simulink subsystem "CtrlEnv_Vehicle_refsub"  (R2023a)
settings: Solver=VariableStepAuto  StartTime=0.0  StopTime=10.0  RelTol=1e-3
undefined symbols (not defined in the file): bevPlant, initial
libraries: fl_lib x28, nesl_utility x11, sdl_lib x1
settings Model: Creator=isaacito  LastModifiedBy=antaeug
settings OptimizationCC: ReuseModelBlockBuffer=off

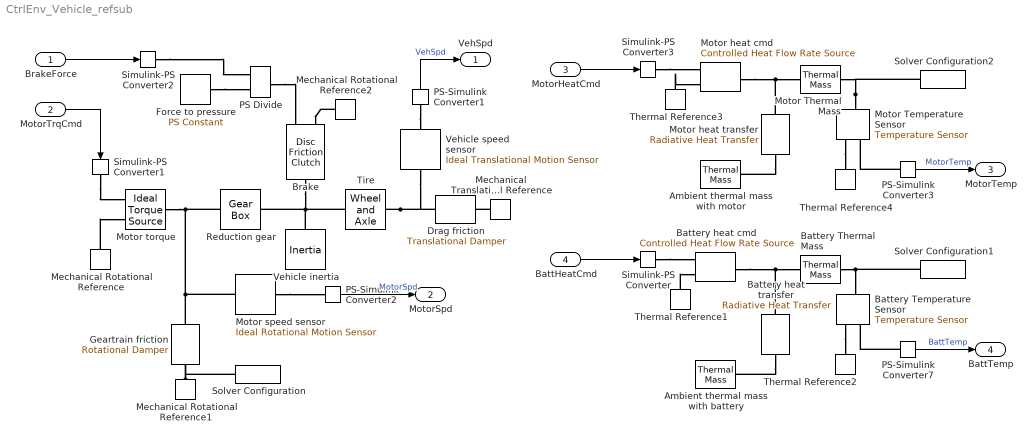
== system CtrlEnv_Vehicle_refsub ==
  BrakeForce : Inport
  MotorTrqCmd : Inport  Port=2
  MotorHeatCmd : Inport  Port=3
  BattHeatCmd : Inport  Port=4
  Ambient thermal mass with battery : fl_lib/Thermal/Thermal Elements/Thermal Mass  mass_type=foundation.enum.constant_variable.constant  mass=1000 t  sp_heat=1000 J/(K*kg)  mass_min=1e-6 kg  num_ports=foundation.enum.numPorts2.one  m_specify=off  m_priority=High  m=1 kg  m_nominal_specify=off  m_nominal_unit=kg  m_nominal_value=1  T_specify=on  T_priority=High  T=initial.BatteryAmbientTemperature_K K  T_nominal_specify=off  T_nominal_unit=K  T_nominal_value=1  Q_specify=off  Q_priority=None  Q=0 W  Q_nominal_specify=off  Q_nominal_unit=W  Q_nominal_value=1
  Ambient thermal mass with motor : fl_lib/Thermal/Thermal Elements/Thermal Mass  mass_type=foundation.enum.constant_variable.constant  mass=1000 t  sp_heat=1000 J/(K*kg)  mass_min=1e-6 kg  num_ports=foundation.enum.numPorts2.one  m_specify=off  m_priority=High  m=1 kg  m_nominal_specify=off  m_nominal_unit=kg  m_nominal_value=1  T_specify=on  T_priority=High  T=initial.MotorAmbientTemperature_K K  T_nominal_specify=off  T_nominal_unit=K  T_nominal_value=1  Q_specify=off  Q_priority=None  Q=0 W  Q_nominal_specify=off  Q_nominal_unit=W  Q_nominal_value=1
  Battery Temperature Sensor : fl_lib/Thermal/Thermal Sensors/Temperature Sensor  temperature_measure=foundation.enum.MeasurementReference.difference
  Battery Thermal Mass : fl_lib/Thermal/Thermal Elements/Thermal Mass  mass_type=foundation.enum.constant_variable.constant  mass=bevPlant.BatteryThermalMass_kg kg  sp_heat=bevPlant.BatterySpecificHeat_J_per_K_per_kg J/(K*kg)  mass_min=1e-6 kg  num_ports=foundation.enum.numPorts2.two  m_specify=off  m_priority=High  m=1 kg  m_nominal_specify=off  m_nominal_unit=kg  m_nominal_value=1  T_specify=on  T_priority=High  T=initial.BatteryTemperature_K K  T_nominal_specify=off  T_nominal_unit=K  T_nominal_value=1  Q_specify=off  Q_priority=None  Q=0 W  Q_nominal_specify=off  Q_nominal_unit=W  Q_nominal_value=1
      settings: InternalSimscapePortConfiguration="{\"Bottom\":[],\"Left\":[{\"id\":\"M\",\"label\":\"\",\"type\":\"foundation.thermal.thermal\"}],\"Right\":[{\"id\":\"N\",\"label\":\"\",\"type\":\"foundation.thermal.thermal\"}],\"Top\":[]}"
  Battery heat cmd : fl_lib/Thermal/Thermal Sources/Controlled Heat Flow Rate Source
  Battery heat transfer : fl_lib/Thermal/Thermal Elements/Radiative Heat Transfer  area=10 m^2  rad_tr_coeff=4e-8 W/(K^4*m^2)  T_specify=off  T_priority=None  T=0 K  T_nominal_specify=off  T_nominal_unit=K  T_nominal_value=1  Q_specify=off  Q_priority=None  Q=0 W  Q_nominal_specify=off  Q_nominal_unit=W  Q_nominal_value=1
      settings: InternalSimscapePortConfiguration="{\"Bottom\":[],\"Left\":[{\"id\":\"A\",\"label\":\"A\",\"type\":\"foundation.thermal.thermal\"}],\"Right\":[{\"id\":\"B\",\"label\":\"B\",\"type\":\"foundation.thermal.thermal\"}],\"Top\":[]}"
  Brake : sdl_lib/Clutches/Disc Friction Clutch  geometry_model=sdl.enum.friction_geometry.radius  r_eff=200 mm  d_o=150 mm  d_i=100 mm  nS=8  piston_area=1 m^2  unidirectional=sdl.enum.directionality.bidirectional  friction_model=sdl.enum.friction_model_TLU_thermal.fixed  mu_w_vector=[0, 100, 1000] rad/s  temperature_TLU=[280, 300, 320] K  mu_static=0.35  mu_static_vector=[.4, .38, .36]  mu_coulomb=0.3  mu_coulomb_vector=[.3, .22, .19]  mu_coulomb_temp_vector=[.3, .28, .25]  mu_coulomb_matrix=[.34, .32, .3; .3, .28, .25; .25, .2, .15]  mu_interp_method=simscape.enum.interpolation.linear  mu_extrap_method=simscape.enum.extrapolation.linear  d_f=1  w_tol=0.001 rad/s  pressure_min=1 Pa  mu_visc=0 N*m*s/rad  initial_state_locked=sdl.enum.initial_lock.unlocked  enable_faults=simscape.enum.onoff.off  fault_type=sdl.enum.clutchFault.lock  external_fault=simscape.enum.onoff.off  temporal_fault=simscape.enum.onoff.off  fault_time=5 s  report_fault=simscape.enum.assert.action.none  thermal_mass=50 kJ/K  T_init=300 K
      settings: InternalSimscapePortConfiguration="{\"Bottom\":[],\"Left\":[{\"id\":\"P\",\"label\":\"P\",\"type\":\"input\"},{\"id\":\"B\",\"label\":\"B\",\"type\":\"foundation.mechanical.rotational.rotational\"}],\"Right\":[{\"id\":\"F\",\"label\":\"F\",\"type\":\"foundation.mechanical.rotational.rotational\"}],\"Top\":[]}"
  Drag friction : fl_lib/Mechanical/Translational Elements/Translational Damper  D=10 N/kph  v_specify=off  v_priority=None  v=0 m/s  v_nominal_specify=off  v_nominal_unit=m/s  v_nominal_value=1  f_specify=off  f_priority=None  f=0 N  f_nominal_specify=off  f_nominal_unit=N  f_nominal_value=1
  Force to pressure : fl_lib/Physical Signals/Sources/PS Constant  constant=1 m^2
  Geartrain friction : fl_lib/Mechanical/Rotational Elements/Rotational Damper  D=0.001 N*m/rpm  w_specify=off  w_priority=None  w=0 rad/s  w_nominal_specify=off  w_nominal_unit=rad/s  w_nominal_value=1  t_specify=off  t_priority=None  t=0 N*m  t_nominal_specify=off  t_nominal_unit=N*m  t_nominal_value=1
  Mechanical Rotational Reference : fl_lib/Mechanical/Rotational Elements/Mechanical Rotational Reference
  Mechanical Rotational Reference1 : fl_lib/Mechanical/Rotational Elements/Mechanical Rotational Reference
  Mechanical Rotational Reference2 : fl_lib/Mechanical/Rotational Elements/Mechanical Rotational Reference
  Mechanical Translational Reference : fl_lib/Mechanical/Translational Elements/Mechanical Translational Reference
  Motor Temperature Sensor : fl_lib/Thermal/Thermal Sensors/Temperature Sensor  temperature_measure=foundation.enum.MeasurementReference.difference
  Motor Thermal Mass : fl_lib/Thermal/Thermal Elements/Thermal Mass  mass_type=foundation.enum.constant_variable.constant  mass=bevPlant.MotorThermalMass_kg kg  sp_heat=bevPlant.MotorSpecificHeat_J_per_K_per_kg J/(K*kg)  mass_min=1e-6 kg  num_ports=foundation.enum.numPorts2.two  m_specify=off  m_priority=High  m=1 kg  m_nominal_specify=off  m_nominal_unit=kg  m_nominal_value=1  T_specify=on  T_priority=High  T=initial.MotorTemperature_K K  T_nominal_specify=off  T_nominal_unit=K  T_nominal_value=1  Q_specify=off  Q_priority=None  Q=0 W  Q_nominal_specify=off  Q_nominal_unit=W  Q_nominal_value=1
      settings: InternalSimscapePortConfiguration="{\"Bottom\":[],\"Left\":[{\"id\":\"M\",\"label\":\"\",\"type\":\"foundation.thermal.thermal\"}],\"Right\":[{\"id\":\"N\",\"label\":\"\",\"type\":\"foundation.thermal.thermal\"}],\"Top\":[]}"
  Motor heat cmd : fl_lib/Thermal/Thermal Sources/Controlled Heat Flow Rate Source
  Motor heat transfer : fl_lib/Thermal/Thermal Elements/Radiative Heat Transfer  area=1 m^2  rad_tr_coeff=4e-8 W/(K^4*m^2)  T_specify=off  T_priority=None  T=0 K  T_nominal_specify=off  T_nominal_unit=K  T_nominal_value=1  Q_specify=off  Q_priority=None  Q=0 W  Q_nominal_specify=off  Q_nominal_unit=W  Q_nominal_value=1
      settings: InternalSimscapePortConfiguration="{\"Bottom\":[],\"Left\":[{\"id\":\"A\",\"label\":\"A\",\"type\":\"foundation.thermal.thermal\"}],\"Right\":[{\"id\":\"B\",\"label\":\"B\",\"type\":\"foundation.thermal.thermal\"}],\"Top\":[]}"
  Motor speed sensor : fl_lib/Mechanical/Mechanical Sensors/Ideal Rotational Motion Sensor  reference=foundation.enum.MeasurementReference.absolute  acceleration_port=false  velocity_port=true  position_port=false  wrap_angle=false  offset=0 rad
      settings: InternalSimscapePortConfiguration="{\"Bottom\":[],\"Left\":[{\"id\":\"R\",\"label\":\"R\",\"type\":\"foundation.mechanical.rotational.rotational\"}],\"Right\":[{\"id\":\"W\",\"label\":\"W\",\"type\":\"output\"}],\"Top\":[]}"
  Motor torque : fl_lib/Mechanical/Mechanical Sources/Ideal Torque Source
  PS Divide : fl_lib/Physical Signals/Functions/PS Divide
  PS-Simulink Converter1 : nesl_utility/PS-Simulink Converter  PhysicalDomain=network_engine_domain  SubClassName=ps_output  LeftPortType=input  RightPortType=output  PseudoPeriodic=off  Frequencies=[]  VectorFormat=inherit  Unit=km/hr  AffineConversion=off
  PS-Simulink Converter2 : nesl_utility/PS-Simulink Converter  PhysicalDomain=network_engine_domain  SubClassName=ps_output  LeftPortType=input  RightPortType=output  PseudoPeriodic=off  Frequencies=[]  VectorFormat=inherit  Unit=rpm  AffineConversion=off
  PS-Simulink Converter3 : nesl_utility/PS-Simulink Converter  PhysicalDomain=network_engine_domain  SubClassName=ps_output  LeftPortType=input  RightPortType=output  PseudoPeriodic=off  Frequencies=[]  VectorFormat=inherit  Unit=degC  AffineConversion=on
  PS-Simulink Converter7 : nesl_utility/PS-Simulink Converter  PhysicalDomain=network_engine_domain  SubClassName=ps_output  LeftPortType=input  RightPortType=output  PseudoPeriodic=off  Frequencies=[]  VectorFormat=inherit  Unit=degC  AffineConversion=on
  Reduction gear : fl_lib/Mechanical/Mechanisms/Gear Box  ratio=bevPlant.ReductionGearRaio  t_in_specify=off  t_in_priority=None  t_in=0 N*m  t_in_nominal_specify=off  t_in_nominal_unit=N*m  t_in_nominal_value=1  t_out_specify=off  t_out_priority=None  t_out=0 N*m  t_out_nominal_specify=off  t_out_nominal_unit=N*m  t_out_nominal_value=1
  Simulink-PS Converter : nesl_utility/Simulink-PS Converter  PhysicalDomain=network_engine_domain  SubClassName=ps_input  LeftPortType=input  RightPortType=output  PseudoPeriodic=off  Frequencies=[]  NoiseDistribution=none  NoiseParameters=[]  Unit=W  AffineConversion=off  FilteringAndDerivatives=provide  SimscapeFilterOrder=1  InputFilterTimeConstant=0.001  UdotUserProvided=0
  Simulink-PS Converter1 : nesl_utility/Simulink-PS Converter  PhysicalDomain=network_engine_domain  SubClassName=ps_input  LeftPortType=input  RightPortType=output  PseudoPeriodic=off  Frequencies=[]  NoiseDistribution=none  NoiseParameters=[]  Unit=N*m  AffineConversion=off  FilteringAndDerivatives=filter  SimscapeFilterOrder=1  InputFilterTimeConstant=0.001  UdotUserProvided=0
  Simulink-PS Converter2 : nesl_utility/Simulink-PS Converter  PhysicalDomain=network_engine_domain  SubClassName=ps_input  LeftPortType=input  RightPortType=output  PseudoPeriodic=off  Frequencies=[]  NoiseDistribution=none  NoiseParameters=[]  Unit=N  AffineConversion=off  FilteringAndDerivatives=provide  SimscapeFilterOrder=1  InputFilterTimeConstant=0.001  UdotUserProvided=0
  Simulink-PS Converter3 : nesl_utility/Simulink-PS Converter  PhysicalDomain=network_engine_domain  SubClassName=ps_input  LeftPortType=input  RightPortType=output  PseudoPeriodic=off  Frequencies=[]  NoiseDistribution=none  NoiseParameters=[]  Unit=W  AffineConversion=off  FilteringAndDerivatives=provide  SimscapeFilterOrder=1  InputFilterTimeConstant=0.001  UdotUserProvided=0
  Solver Configuration : nesl_utility/Solver Configuration  PhysicalDomain=network_engine_domain  SubClassName=solver  LeftPortType=input  RightPortType=generic  Tones=[]  Harmonics=[]  SimulateNoise=off  Profile=off  UseLocalSampling=off  EnableSwitchedLinearOptims=on  FrequencyDomain=off  UseCCode=off  RelTol=0.001  AbsTol=0.001  MinStep=1e-09  ToWorkspace=off  RevertToSquareIcSolve=off  NumHomotopyIterations=100  PhasorMode=off  PhasorModeNumHarmonics=1  ConsistencySolver=NEWTON_XTOL_AFTER_FTOL  IndexReductionMethod=DerivativeReplacement  DoDC=off  ResidualTolerance=1e-09  ConsistencyTolSource=GLOBAL  ConsistencyAbsTol=0.001  ConsistencyRelTol=0.001  ConsistencyTolFactor=0.001  UseLocalSolver=off  LocalSolverChoice=NE_BACKWARD_EULER_ADVANCER  ResolveIndetEquations=on  FunctionEvalNumThread=1  LocalSolverSampleTime=0.001  DoFixedCost=off  MaxNonlinIter=3  MaxModeIter=2  ComputeImpulses=off  ImpulseIterations=2  LinearAlgebra=auto  LinearAlgebraNumThread=0  EquationFormulation=NE_TIME_EF  DelaysMemoryBudget=1024  AutomaticFiltering=on  FilteringTimeConstant=0.001  PartitionStorageMethod=AS_NEEDED  PartitionMemoryBudget=1024  PartitionMethod=ROBUST
      settings: AttributesFormatString=Local solver: %<UseLocalSolver>
  Solver Configuration1 : nesl_utility/Solver Configuration  PhysicalDomain=network_engine_domain  SubClassName=solver  LeftPortType=input  RightPortType=generic  Tones=[]  Harmonics=[]  SimulateNoise=off  Profile=off  UseLocalSampling=off  EnableSwitchedLinearOptims=on  FrequencyDomain=off  UseCCode=off  RelTol=0.001  AbsTol=0.001  MinStep=1e-09  ToWorkspace=off  RevertToSquareIcSolve=off  NumHomotopyIterations=100  PhasorMode=off  PhasorModeNumHarmonics=1  ConsistencySolver=NEWTON_XTOL_AFTER_FTOL  IndexReductionMethod=DerivativeReplacement  DoDC=off  ResidualTolerance=1e-09  ConsistencyTolSource=GLOBAL  ConsistencyAbsTol=0.001  ConsistencyRelTol=0.001  ConsistencyTolFactor=0.001  UseLocalSolver=off  LocalSolverChoice=NE_BACKWARD_EULER_ADVANCER  ResolveIndetEquations=on  FunctionEvalNumThread=1  LocalSolverSampleTime=0.001  DoFixedCost=off  MaxNonlinIter=3  MaxModeIter=2  ComputeImpulses=off  ImpulseIterations=2  LinearAlgebra=auto  LinearAlgebraNumThread=0  EquationFormulation=NE_TIME_EF  DelaysMemoryBudget=1024  AutomaticFiltering=on  FilteringTimeConstant=0.001  PartitionStorageMethod=AS_NEEDED  PartitionMemoryBudget=1024  PartitionMethod=ROBUST
      settings: AttributesFormatString=Local solver: %<UseLocalSolver>
  Solver Configuration2 : nesl_utility/Solver Configuration  PhysicalDomain=network_engine_domain  SubClassName=solver  LeftPortType=input  RightPortType=generic  Tones=[]  Harmonics=[]  SimulateNoise=off  Profile=off  UseLocalSampling=off  EnableSwitchedLinearOptims=on  FrequencyDomain=off  UseCCode=off  RelTol=0.001  AbsTol=0.001  MinStep=1e-09  ToWorkspace=off  RevertToSquareIcSolve=off  NumHomotopyIterations=100  PhasorMode=off  PhasorModeNumHarmonics=1  ConsistencySolver=NEWTON_XTOL_AFTER_FTOL  IndexReductionMethod=DerivativeReplacement  DoDC=off  ResidualTolerance=1e-09  ConsistencyTolSource=GLOBAL  ConsistencyAbsTol=0.001  ConsistencyRelTol=0.001  ConsistencyTolFactor=0.001  UseLocalSolver=off  LocalSolverChoice=NE_BACKWARD_EULER_ADVANCER  ResolveIndetEquations=on  FunctionEvalNumThread=1  LocalSolverSampleTime=0.001  DoFixedCost=off  MaxNonlinIter=3  MaxModeIter=2  ComputeImpulses=off  ImpulseIterations=2  LinearAlgebra=auto  LinearAlgebraNumThread=0  EquationFormulation=NE_TIME_EF  DelaysMemoryBudget=1024  AutomaticFiltering=on  FilteringTimeConstant=0.001  PartitionStorageMethod=AS_NEEDED  PartitionMemoryBudget=1024  PartitionMethod=ROBUST
      settings: AttributesFormatString=Local solver: %<UseLocalSolver>
  Thermal Reference{1..4} (4 alike) : fl_lib/Thermal/Thermal Elements/Thermal Reference
  Tire : fl_lib/Mechanical/Mechanisms/Wheel and Axle  R=bevPlant.TireRollingRadius_m m  or=1  t_specify=off  t_priority=None  t=0 N*m  t_nominal_specify=off  t_nominal_unit=N*m  t_nominal_value=1  f_specify=off  f_priority=None  f=0 N  f_nominal_specify=off  f_nominal_unit=N  f_nominal_value=1
  Vehicle inertia : fl_lib/Mechanical/Rotational Elements/Inertia  inertia=bevPlant.VehicleInertia_kg_m2 kg*m^2  num_ports=foundation.enum.numPorts2.one  w_specify=on  w_priority=High  w=initial.vehicleInertiaSpd_rpm rpm  w_nominal_specify=off  w_nominal_unit=rad/s  w_nominal_value=1  t_specify=off  t_priority=None  t=0 N*m  t_nominal_specify=off  t_nominal_unit=N*m  t_nominal_value=1
  Vehicle speed sensor : fl_lib/Mechanical/Mechanical Sensors/Ideal Translational Motion Sensor  reference=foundation.enum.MeasurementReference.absolute  acceleration_port=false  velocity_port=true  position_port=false  offset=0 m
      settings: InternalSimscapePortConfiguration="{\"Bottom\":[],\"Left\":[{\"id\":\"R\",\"label\":\"R\",\"type\":\"foundation.mechanical.translational.translational\"}],\"Right\":[{\"id\":\"V\",\"label\":\"V\",\"type\":\"output\"}],\"Top\":[]}"
  VehSpd : Outport
  MotorSpd : Outport  Port=2
  MotorTemp : Outport  Port=3
  BattTemp : Outport  Port=4
  wires:
  PS-Simulink Converter7/1 -> BattTemp/1  "BattTemp"
  BattHeatCmd/1 -> Simulink-PS Converter/1
  PS-Simulink Converter3/1 -> MotorTemp/1  "MotorTemp"
  MotorHeatCmd/1 -> Simulink-PS Converter3/1
  MotorTrqCmd/1 -> Simulink-PS Converter1/1
  PS-Simulink Converter1/1 -> VehSpd/1  "VehSpd"
  PS-Simulink Converter2/1 -> MotorSpd/1  "MotorSpd"
  BrakeForce/1 -> Simulink-PS Converter2/1
  connections:
  Motor heat transfer/RConn1 -- Motor heat cmd/LConn1 -- Motor Thermal Mass/RConn1
  Battery heat cmd/LConn1 -- Battery Thermal Mass/RConn1 -- Battery heat transfer/RConn1
  Motor Temperature Sensor/LConn1 -- Solver Configuration2/RConn1 -- Motor Thermal Mass/LConn1
  Tire/RConn1 -- Vehicle speed sensor/LConn1 -- Drag friction/LConn1
  Motor speed sensor/LConn1 -- Reduction gear/LConn1 -- Motor torque/LConn1 -- Geartrain friction/LConn1
  Battery Thermal Mass/LConn1 -- Solver Configuration1/RConn1 -- Battery Temperature Sensor/LConn1
  Geartrain friction/RConn1 -- Solver Configuration/RConn1 -- Mechanical Rotational Reference1/LConn1
  Tire/LConn1 -- Vehicle inertia/LConn1 -- Reduction gear/RConn1 -- Brake/RConn1
  Simulink-PS Converter1/RConn1 -- Motor torque/RConn1
  Motor speed sensor/RConn1 -- PS-Simulink Converter2/LConn1
  Motor heat transfer/LConn1 -- Ambient thermal mass with motor/LConn1
  Simulink-PS Converter/RConn1 -- Battery heat cmd/RConn1
  Mechanical Translational Reference/LConn1 -- Drag friction/RConn1
  PS-Simulink Converter7/LConn1 -- Battery Temperature Sensor/RConn2
  Battery heat transfer/LConn1 -- Ambient thermal mass with battery/LConn1
  Mechanical Rotational Reference/LConn1 -- Motor torque/RConn2
  Thermal Reference1/LConn1 -- Battery heat cmd/RConn2
  Battery Temperature Sensor/RConn1 -- Thermal Reference2/LConn1
  PS-Simulink Converter3/LConn1 -- Motor Temperature Sensor/RConn2
  Motor Temperature Sensor/RConn1 -- Thermal Reference4/LConn1
  PS-Simulink Converter1/LConn1 -- Vehicle speed sensor/RConn1
  Thermal Reference3/LConn1 -- Motor heat cmd/RConn2
  Simulink-PS Converter3/RConn1 -- Motor heat cmd/RConn1
  Force to pressure/RConn1 -- PS Divide/LConn2
  PS Divide/RConn1 -- Brake/LConn1
  Mechanical Rotational Reference2/LConn1 -- Brake/LConn2
  Simulink-PS Converter2/RConn1 -- PS Divide/LConn1
